simulink model "rigPeripheralNet"  (R2012b)
settings: Solver=FixedStepDiscrete  StartTime=0.0  StopTime=10.0  FixedStep=0.001  RelTol=1e-3
undefined symbols (not defined in the file): macaddr, modelConstants
libraries: xpcethernetlib x17, dspmtrx3 x6, simulink x5, xpcnetworkbufferlib x4, Lib_FileLogger x1
(part 2 of 2)

== matlab function rigPeripheralNet/Asynch/Asynch - Control/Make UDP Packet/Add UDP Header ==
  data: sourceIP input uint8 size=[1 4]; packet output; destIP input uint8 size=[1 4]; sourcePort input uint16 size=[1 1]; destPort input uint16 size=[1 1]; UDP_data input uint8; UDP_size input uint16 size=[1 1]; length output uint16 size=[1 1]
function [packet, length] = makeUDP(sourceIP, destIP, sourcePort, destPort, UDP_data, UDP_size)
% create UDP packet

% sourceIP and destIP are 1x4 uint8 of the IP (in address order)
% sourcePort and destPort are uint16
% UDP_data is uint8 of 1xN packet data
% UDP_size is uint16 size of UDP_data
%
% NOTE: UDP_size MUST BE EVEN
FFFF = uint16(hex2dec('FFFF'));

protocol = uint8(hex2dec('11'));

length = UDP_size + uint16(8);

length_BE = (typecast(length, 'uint8')); % flip to big endian
length_BE = length_BE(end:-1:1);

sourcePort_BE = (typecast(sourcePort, 'uint8'));
sourcePort_BE = sourcePort_BE(end:-1:1);

destPort_BE   = (typecast(destPort,   'uint8'));
destPort_BE = destPort_BE(end:-1:1);

header = [sourcePort_BE destPort_BE length_BE uint8([0 0])];

pseudoHeader = [sourceIP destIP uint8(0) protocol length_BE];

% header(7:8) = typecast( bitcmp(uint16(sum( typecast(bitcmp([pseudoHeader header UDP_data]), 'uint16') ))), 'uint8');


checksum = FFFF - uint16(mod( uint32(sum( typecast([pseudoHeader header UDP_data], 'uint16') )), uint32(FFFF) ));
header(7:8) = typecast(checksum, 'uint8');

packet = [ header UDP_data ];

== matlab function rigPeripheralNet/Asynch/Asynch - Data/MATLAB Function ==
  data: u input; y output
function y = padData(u)

z = uint8(zeros(1434, 1))';

z(1:length(u)) = u;

y = z';

== matlab function rigPeripheralNet/Asynch/Asynch - Data/Make UDP Packet/Add IP Header ==
  data: sourceIP input uint8 size=[1 4]; packet output uint8; destIP input uint8 size=[1 4]; IP_data input uint8; IP_size input uint16 size=[1 1]; length output uint16 size=[1 1]
function [packet, length] = makeIP(sourceIP, destIP, IP_data, IP_size)
% create IP packet

FFFF = uint16(hex2dec('FFFF'));

version_IHL = uint8(69); % IPv4 and IP header length of 5
ToS = uint8(0); % no QOS on network

length = IP_size + uint16(20); % hardcode header length to 5

length_BE = (typecast(length, 'uint8')); % change to big endian
length_BE = length_BE(end:-1:1);

% counter
persistent ID % identification
if isempty(ID)
    ID = uint16(0);
else
    ID = ID + 1;
end

ff = [ uint8(bin2dec('01000000')) 0 ]; % don't fragment packets

TTL = uint8(10); % ttl to 10 seconds/hops

protocol = uint8(hex2dec('11')); % UDP Protocol


header = [ version_IHL ToS length_BE typecast(ID, 'uint8') ff TTL protocol 0 0 sourceIP destIP];

% header(11:12) = typecast(bitcmp(uint16(sum( typecast(bitcmp(header), 'uint16') ))), 'uint8'); % checksum

checksum = FFFF - uint16(mod( uint32(sum( typecast(header, 'uint16') )), uint32(FFFF) ));
header(11:12) = typecast(checksum, 'uint8');

packet = [ header IP_data ];

== matlab function rigPeripheralNet/Asynch/Asynch - Data/Make UDP Packet/Add UDP Header ==
  data: sourceIP input uint8 size=[1 4]; packet output; destIP input uint8 size=[1 4]; sourcePort input uint16 size=[1 1]; destPort input uint16 size=[1 1]; UDP_data input uint8; UDP_size input uint16 size=[1 1]; length output uint16 size=[1 1]
function [packet, length] = makeUDP(sourceIP, destIP, sourcePort, destPort, UDP_data, UDP_size)
% create UDP packet

% sourceIP and destIP are 1x4 uint8 of the IP (in address order)
% sourcePort and destPort are uint16
% UDP_data is uint8 of 1xN packet data
% UDP_size is uint16 size of UDP_data
%
% NOTE: UDP_size MUST BE EVEN
FFFF = uint16(hex2dec('FFFF'));

protocol = uint8(hex2dec('11'));

length = UDP_size + uint16(8);

length_BE = (typecast(length, 'uint8')); % flip to big endian
length_BE = length_BE(end:-1:1);

sourcePort_BE = (typecast(sourcePort, 'uint8'));
sourcePort_BE = sourcePort_BE(end:-1:1);

destPort_BE   = (typecast(destPort,   'uint8'));
destPort_BE = destPort_BE(end:-1:1);

header = [sourcePort_BE destPort_BE length_BE uint8([0 0])];

pseudoHeader = [sourceIP destIP uint8(0) protocol length_BE];

% header(7:8) = typecast( bitcmp(uint16(sum( typecast(bitcmp([pseudoHeader header UDP_data]), 'uint16') ))), 'uint8');


checksum = FFFF - uint16(mod( uint32(sum( typecast([pseudoHeader header UDP_data], 'uint16') )), uint32(FFFF) ));
header(7:8) = typecast(checksum, 'uint8');

packet = [ header UDP_data ];

== matlab function rigPeripheralNet/getBehaviorPacket ==
  data: laptopData input Bus: peripheralData size=1; behaviorPacketOut output Bus: behaviorPacketBus size=1; robotData input Bus: peripheralData; windowsData input Bus: peripheralData; windowsPC1Data input Bus: peripheralData; mouseData input
function behaviorPacketOut = getBehaviorPacket(laptopData, robotData, windowsData, windowsPC1Data, mouseData)
%#codegen

persistent behaviorPacket;
persistent robotPacket;
persistent windowsPacket;
persistent windowsPC1Packet;
persistent pc1MousePacket;

if isempty(behaviorPacket)
    behaviorPacket = initBehaviorPacket;
end

if isempty(robotPacket)
    robotPacket = initRobotPacket;
end

if isempty(windowsPacket)
    windowsPacket = initWindowsPacket;
end

if isempty(windowsPC1Packet)
    windowsPC1Packet = initWindowsPC1Packet;
end

if isempty(pc1MousePacket)
    pc1MousePacket = initPC1MousePacket;
end

%% ALWAYS PARSE BEHAVIOR PACKETS IF THERE ARE ANY
if laptopData.receive 
    if laptopData.dataLen == 528
        behaviorPacket = parseBehaviorPacket(laptopData.data);
    end
    behaviorPacket.packetSize = laptopData.dataLen;
end

%% ALWAYS PARSE ROBOT PACKETS IF THERE ARE ANY
if robotData.receive 
%     if robotData.dataLen == 48 % 28 for IP + UDP header, 20 for data
    % if robotData.dataLen == 52 % 28 for IP + UDP header, 24 for data
    if robotData.dataLen == 104 % 28 for IP + UDP header, 76 for data
        robotPacket = parseRobotPacket(robotData.data);
    end
    robotPacket.packetSize = robotData.dataLen;

    behaviorPacket.robotTimestamp = robotPacket.robotTimestamp;
    behaviorPacket.robotPosition = robotPacket.robotPosition;
    behaviorPacket.robotDataAge = robotPacket.robotDataAge; % always 0, since not used
    behaviorPacket.robotPacketSize = robotPacket.packetSize; 
end

%% ALWAYS PARSE WINDOWS PACKETS IF THERE ARE ANY
if windowsData.receive 
    if windowsData.dataLen == 64 % should be 28 for IP + UDP header plus 12 for data = 40, but for some reason there are 6 extra
        windowsPacket = parseWindowsPacket(windowsData.data);
    end
    windowsPacket.packetSize = windowsData.dataLen;
    
    behaviorPacket.windowsTimestamp = windowsPacket.windowsTimestamp;
    behaviorPacket.windowsMousePosition = windowsPacket.windowsMousePosition;
    behaviorPacket.rigidBodyPosXYZ = windowsPacket.rigidBodyPosXYZ;
    behaviorPacket.rigidBodyRotXYZ = windowsPacket.rigidBodyRotXYZ;
    behaviorPacket.windowsPacketSize = windowsPacket.packetSize; 
end

%% ALWAYS PARSE WINDOWS PC1 PACKETS IF THERE ARE ANY (eye data for now)
if windowsPC1Data.receive 
    if windowsPC1Data.dataLen == 92 %according to wireshark
        windowsPC1Packet = parseWindowsPC1Packet(windowsPC1Data.data);
    end
    windowsPC1Packet.packetSize = windowsPC1Data.dataLen;

    behaviorPacket.windowsPC1TobiiTimestamp = windowsPC1Packet.windowsPC1TobiiTimestamp;
    behaviorPacket.windowsPC1Timestamp = windowsPC1Packet.windowsPC1Timestamp;
    behaviorPacket.windowsPC1GazePoint = windowsPC1Packet.windowsPC1GazePoint;
    behaviorPacket.windowsPC1GazeValid = windowsPC1Packet.windowsPC1GazeValid; 
    behaviorPacket.windowsPC1HeadPos = windowsPC1Packet.windowsPC1HeadPos;
    behaviorPacket.windowsPC1HeadPosValid = windowsPC1Packet.windowsPC1HeadPosValid;
    behaviorPacket.windowsPC1HeadRot = windowsPC1Packet.windowsPC1HeadRot;
    behaviorPacket.windowsPC1HeadRotValid = windowsPC1Packet.windowsPC1HeadRotValid; 
end

%% ALWAYS PARSE WINDOWS PC1 MOUSE PACKETS IF THERE ARE ANY 
if mouseData.receive 
    if mouseData.dataLen == 46 %according to wireshark
        pc1MousePacket = parsePC1MousePacket(mouseData.data);
    end
    pc1MousePacket.packetSize = mouseData.dataLen;

    behaviorPacket.pc1MouseTimestamp = pc1MousePacket.pc1MouseTimestamp;
    behaviorPacket.pc1MousePos = pc1MousePacket.pc1MousePos;
end

%%
behaviorPacketOut = behaviorPacket;

end

function behaviorPacket = parseBehaviorPacket(packetData)
    behaviorPacket = initBehaviorPacket();
    pointer = 28;
    xrc = typecast(packetData(pointer+[1:4]), 'uint32');
    behaviorPacket.xpcRequestClock = xrc(1);
    
    pointer = pointer+4;
    imang = typecast(packetData(pointer+[1:12]), 'single');
    behaviorPacket.imuAngle(1:3) = imang(1:3);
    
    pointer = pointer+12;
    imacc = typecast(packetData(pointer+[1:12]), 'single');
    behaviorPacket.imuAccel(1:3) = imacc(1:3);
    
    pointer = pointer+12;
    imgyr = typecast(packetData(pointer+[1:12]), 'single');
    behaviorPacket.imuGyro(1:3) = imgyr(1:3);
    
    pointer = pointer+12;
    imcomp = typecast(packetData(pointer+[1:12]), 'single');
    behaviorPacket.imuCompass(1:3) = imcomp(1:3);
    
    pointer = pointer+12;
    imdag = typecast(packetData(pointer+[1:4]), 'single');
    behaviorPacket.imuDataAge(1) = imdag(1);
    
    pointer = pointer+4;
    glv = typecast(packetData(pointer+[1:10]), 'uint16');
    behaviorPacket.glove(1:5) = glv(1:5);

    pointer = pointer+10;
    glda = typecast(packetData(pointer+[1:4]), 'single');
    behaviorPacket.gloveDataAge(1) = glda(1);
    
    pointer = pointer+4;
    glserial = typecast(packetData(pointer+[1:12]), 'uint8');
    behaviorPacket.gloveSerial(1:12) = glserial(1:12);
    
    pointer = pointer+12;
    glv2 = typecast(packetData(pointer+[1:10]), 'uint16');
    behaviorPacket.glove2(1:5) = glv2(1:5);

    pointer = pointer+10;
    glda2 = typecast(packetData(pointer+[1:4]), 'single');
    behaviorPacket.gloveDataAge2(1) = glda2(1);
    
    pointer = pointer+4;
    glserial2 = typecast(packetData(pointer+[1:12]), 'uint8');
    behaviorPacket.gloveSerial2(1:12) = glserial2(1:12);
    
    pointer = pointer+12;
    m = typecast(packetData(pointer+[1:24]), 'int32');
    behaviorPacket.mouse(1:6) = m(1:6);

    pointer = pointer+24;
    mda = typecast(packetData(pointer+[1:4]), 'single');
    behaviorPacket.mouseDataAge(1) = mda(1);

    pointer = pointer+4;
    lts = typecast(packetData(pointer+[1:16]), 'uint8');
    behaviorPacket.peripheralTimestamp(1:16) = lts(1:16);

end

function rPacket = parseRobotPacket(pData)

    rPacket = initRobotPacket();
    pointer = 28;

    robotTimestamp = typecast(pData(pointer+[1:4]), 'single');
    rPacket.robotTimestamp = robotTimestamp;
    pointer = pointer + 4;
    
%     robotPosition = typecast(pData(pointer+[1:12]), 'single');
%     rPacket.robotPosition(1:3) = robotPosition(1:3);
%     pointer = pointer + 12; % 3 4-byte singles
%   SDS Jun 2017  increasing by 1 elemnt
%     robotPosition = typecast(pData(pointer+[1:16]), 'single'); 
%     rPacket.robotPosition(1:4) = robotPosition(1:4);
%     pointer = pointer + 16; % 4 4-byte singles
    
    % SDS Jun 2017  increasing to 18 elements
    robotPosition = typecast(pData(pointer+[1:72]), 'single'); 
    rPacket.robotPosition(1:18) = robotPosition(1:18);
    pointer = pointer + 72; % 18 4-byte singles
        
    % no such thing as data age any more
%     robotDataAge = typecast(pData(pointer+[1:4]), 'single');
%     rPacket.robotDataAge = robotDataAge;
%     pointer = pointer + 4;
    rPacket.robotDataAge = single(0);
end

function wPacket = parseWindowsPacket(pData)
    pointer = 28;
    wPacket = initWindowsPacket();
    
    windowsTimestamp = typecast(pData(pointer+[1:4]), 'single');
    wPacket.windowsTimestamp = windowsTimestamp;
    pointer = pointer + 4;

    windowsMousePosition =  typecast(pData(pointer+[1:8]), 'single'); 
    wPacket.windowsMousePosition(1:2) = windowsMousePosition(1:2);
    pointer = pointer + 8; 
    
    rigidBodyPosXYZ =  typecast(pData(pointer+[1:12]), 'single'); 
    wPacket.rigidBodyPosXYZ(1:3) = rigidBodyPosXYZ(1:3);
    pointer = pointer + 12; 
    
    rigidBodyRotXYZ =  typecast(pData(pointer+[1:12]), 'single'); 
    wPacket.rigidBodyRotXYZ(1:3) = rigidBodyRotXYZ(1:3);
    pointer = pointer + 12; 
end

function wPacket = parsePC1MousePacket(pData)
    pointer = 28;
    wPacket = initPC1MousePacket();
    
    pc1MouseTimestamp = typecast(pData(pointer+[1:4]), 'single');
    wPacket.pc1MouseTimestamp = pc1MouseTimestamp;
    pointer = pointer + 4;

    pc1MousePos =  typecast(pData(pointer+[1:8]), 'single'); 
    wPacket.pc1MousePos(1:2) = pc1MousePos(1:2);
    pointer = pointer + 8; 
end

function wPacket = parseWindowsPC1Packet(pData)
    pointer = 28;
    wPacket = initWindowsPC1Packet();
    
    windowsPC1TobiiTimestamp = typecast(pData(pointer+[1:8]), 'uint32'); %actually a uint64
    wPacket.windowsPC1TobiiTimestamp(1:2) = windowsPC1TobiiTimestamp(1:2);
    pointer = pointer + 8;

    windowsPC1Timestamp =  typecast(pData(pointer+[1:4]), 'uint32'); 
    wPacket.windowsPC1Timestamp = windowsPC1Timestamp;
    pointer = pointer + 4; 
    
    windowsPC1GazePoint =  typecast(pData(pointer+[1:8]), 'single'); 
    wPacket.windowsPC1GazePoint(1:2) = windowsPC1GazePoint(1:2);
    pointer = pointer + 8; 
    
    windowsPC1GazeValid =  typecast(pData(pointer+[1:4]), 'uint32'); 
    wPacket.windowsPC1GazeValid = uint8(windowsPC1GazeValid);
    pointer = pointer + 4; 
    
    windowsPC1HeadPos =  typecast(pData(pointer+[1:12]), 'single'); 
    wPacket.windowsPC1HeadPos(1:3) = windowsPC1HeadPos(1:3);
    pointer = pointer + 12; 
    
    windowsPC1HeadPosValid =  typecast(pData(pointer+[1:4]), 'uint32'); 
    wPacket.windowsPC1HeadPosValid = uint8(windowsPC1HeadPosValid);
    pointer = pointer + 4; 

    windowsPC1HeadRot =  typecast(pData(pointer+[1:12]), 'single'); 
    wPacket.windowsPC1HeadRot(1:3) = windowsPC1HeadRot(1:3);
    pointer = pointer + 12; 
    
    windowsPC1HeadRotValidX =  typecast(pData(pointer+[1:4]), 'uint32'); 
    wPacket.windowsPC1HeadRotValid(1) = uint8(windowsPC1HeadRotValidX);
    pointer = pointer + 4; 
    
    windowsPC1HeadRotValidY =  typecast(pData(pointer+[1:4]), 'uint32'); 
    wPacket.windowsPC1HeadRotValid(2) = uint8(windowsPC1HeadRotValidY);
    pointer = pointer + 4; 
    
    windowsPC1HeadRotValidZ =  typecast(pData(pointer+[1:4]), 'uint32'); 
    wPacket.windowsPC1HeadRotValid(3) = uint8(windowsPC1HeadRotValidZ);
    pointer = pointer + 4; 
end

function behaviorPacket = initBehaviorPacket()

    behaviorPacket.xpcRequestClock = uint32(0);
    behaviorPacket.imuAngle = single(zeros(3,1));
    behaviorPacket.imuAccel = single(zeros(3,1));
    behaviorPacket.imuGyro = single(zeros(3,1));
    behaviorPacket.imuCompass = single(zeros(3,1));
    behaviorPacket.imuDataAge = single(inf);
    behaviorPacket.glove = uint16(zeros(5,1));
    behaviorPacket.gloveDataAge = single(inf);
    behaviorPacket.gloveSerial = uint8(zeros(12,1));
    behaviorPacket.glove2 = uint16(zeros(5,1));
    behaviorPacket.gloveDataAge2 = single(inf);
    behaviorPacket.gloveSerial2 = uint8(zeros(12,1));
    behaviorPacket.mouse = int32(zeros(6,1));
    behaviorPacket.mouseDataAge = single(inf);
    behaviorPacket.peripheralTimestamp = uint8(zeros(16,1));
    behaviorPacket.packetSize = uint16(zeros(1,1));
    behaviorPacket.robotTimestamp = single(0);
%     behaviorPacket.robotPosition = single(zeros(3, 1));
    behaviorPacket.robotPosition = single(zeros(18, 1));
    behaviorPacket.robotDataAge = single(0);
    behaviorPacket.robotPacketSize = uint16(0);
    
    behaviorPacket.windowsTimestamp = single(0);
    behaviorPacket.windowsMousePosition = single(zeros(2,1));
    behaviorPacket.rigidBodyPosXYZ = single(zeros(3,1));
    behaviorPacket.rigidBodyRotXYZ = single(zeros(3,1));
    behaviorPacket.windowsPacketSize = uint16(0);
    
    behaviorPacket.windowsPC1TobiiTimestamp = uint32(zeros(2,1)); %actually a uint64
    behaviorPacket.windowsPC1Timestamp = uint32(0);
    
    behaviorPacket.windowsPC1GazePoint = single(zeros(2,1));
    behaviorPacket.windowsPC1GazeValid = uint8(0);
    
    behaviorPacket.windowsPC1HeadPos = single(zeros(3,1));
    behaviorPacket.windowsPC1HeadPosValid = uint8(0);
    
    behaviorPacket.windowsPC1HeadRot = single(zeros(3,1));
    behaviorPacket.windowsPC1HeadRotValid = uint8(zeros(3,1));
    
    behaviorPacket.pc1MouseTimestamp = single(0);
    behaviorPacket.pc1MousePos =single(zeros(2,1));
end

function rPacket = initRobotPacket()

    rPacket.robotTimestamp = single(zeros(1, 1)); % timestamp
%     rPacket.robotPosition = single(zeros(3, 1)); % x, y z
%     rPacket.robotPosition = single(zeros(4, 1)); % x, y z r1
    % xSet ySet zSet twistSet fanSet gripSet, ...
    % xState yState zState rxState ryState rzState tau1State tau2State
    % tau3State tau4State tau5State tau6State
    rPacket.robotPosition = single(zeros(18, 1)); 
    rPacket.robotDataAge = single(inf);
    rPacket.packetSize = uint16(0);

end

function wPacket = initWindowsPacket()

    wPacket.windowsTimestamp = single(zeros(1, 1)); % timestamp
    wPacket.windowsMousePosition = single(zeros(2, 1)); 
    wPacket.packetSize = uint16(0);
    
    wPacket.rigidBodyPosXYZ = single(zeros(3,1));
    wPacket.rigidBodyRotXYZ =  single(zeros(3,1));
end

function wPacket = initWindowsPC1Packet()

    wPacket.packetSize = uint16(0);

    wPacket.windowsPC1TobiiTimestamp = uint32(zeros(2,1)); %actually a uint64
    wPacket.windowsPC1Timestamp = uint32(0);
    
    wPacket.windowsPC1GazePoint = single(zeros(2,1));
    wPacket.windowsPC1GazeValid = uint8(0);
    
    wPacket.windowsPC1HeadPos = single(zeros(3,1));
    wPacket.windowsPC1HeadPosValid = uint8(0);
    
    wPacket.windowsPC1HeadRot = single(zeros(3,1));
    wPacket.windowsPC1HeadRotValid = uint8(zeros(3,1));
end
    
function wPacket = initPC1MousePacket()

    wPacket.pc1MouseTimestamp = single(zeros(1, 1)); % timestamp
    wPacket.pc1MousePos = single(zeros(2, 1)); 
    wPacket.packetSize = uint16(0);

end
